simulink model "PI_controller"  (R2020a)
settings: Solver=VariableStepAuto  StartTime=0.0  StopTime=10.0  RelTol=1e-3
settings Model: Creator=Ishan's PC  LastModifiedBy=Ishan's PC

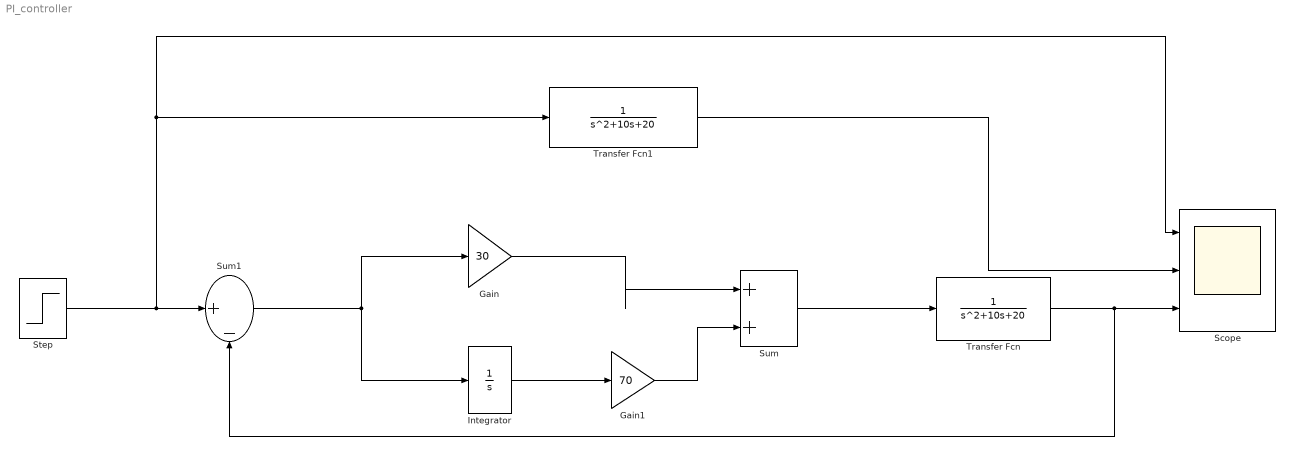
== system PI_controller ==
  Gain : Gain  Gain=30
  Gain1 : Gain  Gain=70
  Integrator : Integrator
  Scope : Scope  NumInputPorts=3
  Step : Step  SampleTime=0
  Sum : Sum  Inputs=|++
  Sum1 : Sum  Inputs=|+-
  Transfer Fcn : TransferFcn  Denominator=[1 10 20]
  Transfer Fcn1 : TransferFcn  Denominator=[1 10 20]
  wires:
  Step/1 -> Transfer Fcn1/1, Scope/1, Sum1/1
  Sum1/1 -> Gain/1, Integrator/1
  Integrator/1 -> Gain1/1
  Gain/1 -> Sum/1
  Gain1/1 -> Sum/2
  Sum/1 -> Transfer Fcn/1
  Transfer Fcn/1 -> Sum1/2, Scope/3
  Transfer Fcn1/1 -> Scope/2
